simulink model "model5_1"  (R2024b)
settings: Solver=VariableStepAuto  StartTime=0.0  StopTime=20  RelTol=1e-3
values from neighbouring files (symbols this model uses):
  R = double(RS(1:n))    [calculateRS.m]
  S = double(RS(n+1:end))    [calculateRS.m]
  T = 1 / dcgain(1/Rs * feedback(Gp, Ss/Rs))    [domaci5.m]    (also in domaci5_1.m)
settings Model: Creator=neso  LastModifiedBy=neso

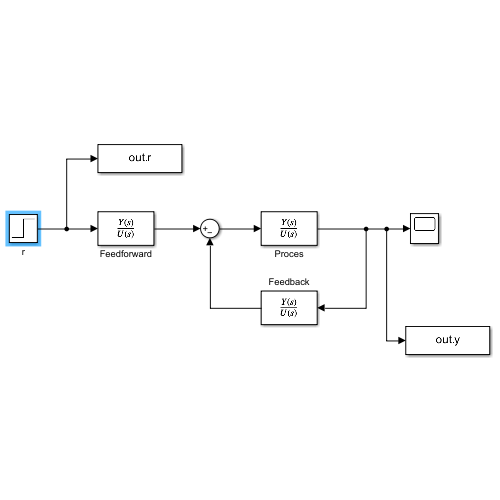
[thumbnail: Simulink's stored preview of the top-level diagram]
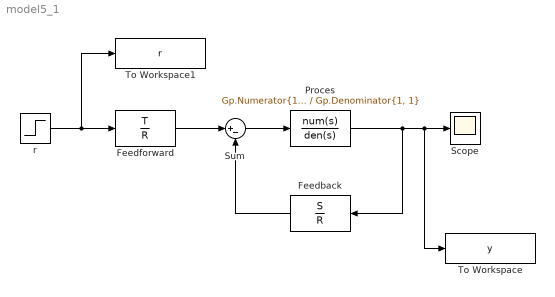
== system model5_1 ==
  Feedback : TransferFcn  Numerator=S  Denominator=R
  Feedforward : TransferFcn  Numerator=T  Denominator=R
  Proces : TransferFcn  Numerator=Gp.Numerator{1, 1}  Denominator=Gp.Denominator{1, 1}
  Scope : Scope
  Sum : Sum  Inputs=|+-
  To Workspace : ToWorkspace  VariableName=y  SaveFormat=Timeseries  SampleTime=-1
  To Workspace1 : ToWorkspace  VariableName=r  SaveFormat=Timeseries  SampleTime=-1
  r : Step  Time=0  After=5  SampleTime=0
  wires:
  Feedforward/1 -> Sum/1
  Sum/1 -> Proces/1
  Feedback/1 -> Sum/2
  r/1 -> To Workspace1/1, Feedforward/1
  Proces/1 -> To Workspace/1, Scope/1, Feedback/1
